simulink model "TEST_LIDAR"  (R2022b)
settings: Solver=FixedStepAuto  StartTime=0.0  StopTime=inf  FixedStep=1e-3  RelTol=1e-3  EnableMultiTasking=on
model workspace (MAT data in the model file):
  SL_ROS_VariableLengthArrays_MaxSizes : object (value not decoded)
values from neighbouring files (symbols this model uses):
  data = theClient.GetLastFrameOfData()    [FuncMotive.m]
undefined symbols (not defined in the file or in its folder): angular, carstamp, CIRCUIT, CLTF_DAMP, CLTF_FREQ, CLTF_GAIN, CONTROL, CONTROL_INI, DiscIntNeverNeededParam, INPUT, linear, MCP3201, MD25, MODEL, MODEL_INI, mpcstate, MPU60X0, MPU9250, MSG, NAV_MPC_CONTROL, OUTPUT, RCRX, SAMPLING_TIME, SYSID_INPUT, VL6180X
libraries: raspberrypiCommlib x160, simulink x89, raspberrypiNetworklib x22, ros2lib x14, dspsigattribs x14, embedlinuxBasiclib x12, ctrlSharedLib x2, mpclib x1, vrlib x1, sldrtlib x1
(part 15 of 19)

== matlab function TEST_LIDAR/SIMULATION/RC TRANSMITTER /BUS UPDATE ==
  data: CONTROL_IN input; CONTROL output Bus: CONTROL_Bus; CH_RAW input size=14
function CONTROL = RCRX_UPDATE(CONTROL_IN,CH_RAW)
%--------------------------------------------------------------
% COPY CONTROL BUS
CONTROL = CONTROL_IN;
%--------------------------------------------------------------
% SCALING PARAMETERS
% Open-loop RC scale {'COM MOTOR VOLT','DIFF MOTOR VOLT'}
OPL_RC_SCALE = CONTROL.PARAM.OPL_RC_SCALE;
% Velocity RC scale {'FORWARD VEL REF','YAW RATE REF'}
VEL_RC_SCALE = CONTROL.PARAM.VEL_RC_SCALE;
% Wall follower RC scale {'FORWARD VEL REF','WALL DIST REF'}
WFL_RC_SCALE = CONTROL.PARAM.WFL_RC_SCALE;
% Navigation RC scale {'INC POS X REF','INC POS Y REF'}
NAV_RC_SCALE = CONTROL.PARAM.NAV_RC_SCALE;
%--------------------------------------------------------------
% CHANNEL CALIBRATION
CALIB_PARAM = CONTROL.PARAM.RC_CALIB_PARAM;
CH_TRIM = CONTROL.PARAM.RC_CH_TRIM;
NUM_CH = length(CH_RAW);
CH_PU = zeros(NUM_CH,1);
CH_RAW = double(CH_RAW);
for nn = 1:NUM_CH
    CH_PU(nn) = (CALIB_PARAM(nn,1)*CH_RAW(nn) + CALIB_PARAM(nn,2)).*double(CH_RAW(nn)<CH_TRIM(nn)) + ...
                (CALIB_PARAM(nn,3)*CH_RAW(nn) + CALIB_PARAM(nn,4)).*double(CH_RAW(nn)>=CH_TRIM(nn));
end        
% Channel definition : {'COM MOTOR VOLT','DIFF MOTOR VOLT'}
%                      {'FORWARD VEL REF','YAW RATE REF'}
%                      {'FORWARD VEL REF','YAW ANGLE REF'}
%                      {'FORWARD VEL REF','WALL DIST REF'}
%                      {'INC POS X REF','INC POS Y REF'}
CH_DEF = CONTROL.PARAM.RC_CH_DEF;
% Throttle channel between 0 and 1 
% CH_PU(CH_DEF(4)) = (CH_PU(CH_DEF(4))+1)/2; 
%--------------------------------------------------------------
% TARGET DEFINITION
switch CONTROL.STATE.CONTROL_MODE 
    case 0 % OPEN LOOP
        % {'COMMON MOTOR VOLT','DIFFERENTIAL MOTOR VOLT'}
        if CONTROL.STATE.MV_TARGET_SOURCE(1)==2 % JOYSTICK
            CONTROL.TARGET.MOTOR_VOLT_CD_REF_RC(1) = CH_PU(CH_DEF(1))*OPL_RC_SCALE(1);
        end
        if CONTROL.STATE.MV_TARGET_SOURCE(2)==2 % JOYSTICK
            CONTROL.TARGET.MOTOR_VOLT_CD_REF_RC(2) = CH_PU(CH_DEF(2))*OPL_RC_SCALE(2);
        end
        if CONTROL.STATE.MV_TARGET_SOURCE(1)==3 % SWITCH
            CONTROL.TARGET.MOTOR_VOLT_CD_REF_RC(1) = CONTROL.PARAM.OPL_RC_SWITCH(1,round(2+CH_PU(5)));
        end
        if CONTROL.STATE.MV_TARGET_SOURCE(2)==3 % SWITCH
            CONTROL.TARGET.MOTOR_VOLT_CD_REF_RC(2) = CONTROL.PARAM.OPL_RC_SWITCH(2,round(2+CH_PU(6)));
        end       
    case 1 % FORWARD VELOCITY AND YAW ANGLE
        % {'FORWARD VEL REF','YAW ANGLE REF'}
        if CONTROL.STATE.FV_TARGET_SOURCE==2 % JOYSTICK
            CONTROL.TARGET.FORWARD_VEL_REF_RC = CH_PU(CH_DEF(1))*VEL_RC_SCALE(1);
        end
        if CONTROL.STATE.YA_TARGET_SOURCE==2 % JOYSTICK
            CONTROL.TARGET.YAW_ANG_REF_RC = CH_PU(CH_DEF(2))*VEL_RC_SCALE(2);
        end
        if CONTROL.STATE.FV_TARGET_SOURCE==3 % SWITCH
            CONTROL.TARGET.FORWARD_VEL_REF_RC = CONTROL.PARAM.VEL_RC_SWITCH(1,round(2+CH_PU(5)));
        end
        if CONTROL.STATE.YA_TARGET_SOURCE==3 % SWITCH
            CONTROL.TARGET.YAW_ANG_REF_RC = CONTROL.PARAM.VEL_RC_SWITCH(2,round(2+CH_PU(6)));
        end
    case 2 % FORWARD VELOCITY AND YAW RATE
        % {'FORWARD VEL REF','YAW RATE REF'}
        if CONTROL.STATE.FV_TARGET_SOURCE==2 % JOYSTICK
            CONTROL.TARGET.FORWARD_VEL_REF_RC = CH_PU(CH_DEF(1))*VEL_RC_SCALE(1);
        end
        if CONTROL.STATE.YR_TARGET_SOURCE==2 % JOYSTICK
            CONTROL.TARGET.YAW_RATE_REF_RC = CH_PU(CH_DEF(2))*VEL_RC_SCALE(2);
        end
        if CONTROL.STATE.FV_TARGET_SOURCE==3 % SWITCH
            CONTROL.TARGET.FORWARD_VEL_REF_RC = CONTROL.PARAM.VEL_RC_SWITCH(1,round(2+CH_PU(5)));
        end
        if CONTROL.STATE.YR_TARGET_SOURCE==3 % SWITCH
            CONTROL.TARGET.YAW_RATE_REF_RC = CONTROL.PARAM.VEL_RC_SWITCH(2,round(2+CH_PU(6)));
        end
    case 3 % NAVIGATION
        % {'INC POS X REF','INC POS Y REF'}
        if CONTROL.STATE.NAV_TARGET_SOURCE==2 % JOYSTICK
            CONTROL.TARGET.NAV_REF_RC(1) = CONTROL.INPUT.NAV_MO(1) + CH_PU(CH_DEF(1))*NAV_RC_SCALE;
            CONTROL.TARGET.NAV_REF_RC(2) = CONTROL.INPUT.NAV_MO(2) + CH_PU(CH_DEF(1))*NAV_RC_SCALE;
        end
        if CONTROL.STATE.NAV_TARGET_SOURCE==3 % SWITCH
            % CONTROL.TARGET.NAV_REF_RC(1) = CONTROL.INPUT.NAV_MO(1) + CONTROL.PARAM.NAV_RC_SWITCH(1,round(2+CH_PU(5)));
            % CONTROL.TARGET.NAV_REF_RC(2) = CONTROL.INPUT.NAV_MO(2) + CONTROL.PARAM.NAV_RC_SWITCH(2,round(2+CH_PU(6)));
            CONTROL.TARGET.NAV_REF_RC(1) = CONTROL.PARAM.NAV_RC_SWITCH(1,round(2+CH_PU(5)));
            CONTROL.TARGET.NAV_REF_RC(2) = CONTROL.PARAM.NAV_RC_SWITCH(2,round(2+CH_PU(6)));
        end
    case {4,5} % WALL FOLLOWER
        % {'FORWARD VEL REF','WALL DIST REF'}
        if CONTROL.STATE.FV_TARGET_SOURCE==2 % JOYSTICK
            CONTROL.TARGET.FORWARD_VEL_REF_RC = CH_PU(CH_DEF(1))*WFL_RC_SCALE(1);
        end
        % {'FORWARD VEL REF','WALL DIST REF'}
        if CONTROL.STATE.WD_TARGET_SOURCE==2 % JOYSTICK
            CONTROL.TARGET.WALL_DIST_REF_RC = 0.1 + CH_PU(CH_DEF(2))*WFL_RC_SCALE(2);
        end
        if CONTROL.STATE.FV_TARGET_SOURCE==3 % SWITCH
            CONTROL.TARGET.FORWARD_VEL_REF_RC = CONTROL.PARAM.WFL_RC_SWITCH(1,round(2+CH_PU(5)));
        end
        if CONTROL.STATE.WD_TARGET_SOURCE==3 % SWITCH
            CONTROL.TARGET.WALL_DIST_REF_RC = CONTROL.PARAM.WFL_RC_SWITCH(2,round(2+CH_PU(6)));
        end
    otherwise % FORWARD VELOCITY AND YAW RATE
        % {'FORWARD VEL REF','YAW RATE REF'}
        if CONTROL.STATE.FV_TARGET_SOURCE==2 % JOYSTICK
            CONTROL.TARGET.FORWARD_VEL_REF_RC = CH_PU(CH_DEF(1))*VEL_RC_SCALE(1);
        end
        if CONTROL.STATE.YR_TARGET_SOURCE==2 % JOYSTICK
            CONTROL.TARGET.YAW_RATE_REF_RC = CH_PU(CH_DEF(2))*VEL_RC_SCALE(1);
        end
        if CONTROL.STATE.FV_TARGET_SOURCE==3 % SWITCH
            CONTROL.TARGET.FORWARD_VEL_REF_RC = CONTROL.PARAM.VEL_RC_SWITCH(1,round(2+CH_PU(5)));
        end
        if CONTROL.STATE.YR_TARGET_SOURCE==3 % SWITCH
            CONTROL.TARGET.YAW_RATE_REF_RC = CONTROL.PARAM.VEL_RC_SWITCH(2,round(2+CH_PU(6)));
        end
end
if abs(CONTROL.TARGET.MOTOR_VOLT_CD_REF_RC(1))<0.25
    CONTROL.TARGET.MOTOR_VOLT_CD_REF_RC(1) = 0;
end
if abs(CONTROL.TARGET.MOTOR_VOLT_CD_REF_RC(2))<0.25
    CONTROL.TARGET.MOTOR_VOLT_CD_REF_RC(2) = 0;
end
if abs(CONTROL.TARGET.FORWARD_VEL_REF_RC)<0.05
    CONTROL.TARGET.FORWARD_VEL_REF_RC = 0;
end
if abs(CONTROL.TARGET.YAW_RATE_REF_RC)<0.025
    CONTROL.TARGET.YAW_RATE_REF_RC = 0;
end
%--------------------------------------------------------------
% CONTROL BUS UPDATE
% RC CHANNELS (pu): channel range [-1 1] / Throtle range (channel 4) [0 1] 
CONTROL.TARGET.RC_CH_PU = CH_PU(:);
CONTROL.TARGET.RC_CH_RAW = CH_RAW(:);

== matlab function TEST_LIDAR/HARDWARE/SENSORS/IMU MPU60X0_SPI/READ IMU/GRAVITY ROTATION ==
  data: PITCH_OFFSET input; GRAVITY_VECTOR output; GRAVITY input; VEHICLE_MODE input
function GRAVITY_VECTOR = GRAVITY_ROTATION(PITCH_OFFSET,GRAVITY,VEHICLE_MODE)
if VEHICLE_MODE
    ROTATION_MATRIX = [cos(PITCH_OFFSET) 0 -sin(PITCH_OFFSET) ; 0 1 0 ; sin(PITCH_OFFSET) 0 cos(PITCH_OFFSET)];
    GRAVITY_VECTOR = ROTATION_MATRIX*[GRAVITY ; 0 ; 0];
else
    GRAVITY_VECTOR = [0 ; 0 ; -GRAVITY];
end

== matlab function TEST_LIDAR/SIMULATION/READ ENCODER/READ_ENCODER ==
  data: MODEL input Bus: MODEL_Bus; CONTROL_IN input Bus: CONTROL_Bus; CONTROL output Bus: CONTROL_Bus
function CONTROL = READ_ENCODER(MODEL,CONTROL_IN)

%--------------------------------------------------------------
% UPDATE BUS
%--------------------------------------------------------------
CONTROL = CONTROL_IN;

%--------------------------------------------------------------
% STATE
%--------------------------------------------------------------
persistent initialize left_enc_prv right_enc_prv inc_com_ang_prv ...
           inc_dif_ang_prv inc2_com_ang_prv inc2_dif_ang_prv dif_ang ...
           dif_ang_offs left_enc_offs right_enc_offs ENC_ANG

if isempty(initialize)
    left_enc_prv = zeros(2,1);
    right_enc_prv = zeros(2,1);
    left_enc_offs = 0;
    right_enc_offs = 0;
    inc_com_ang_prv = zeros(5,1);
    inc_dif_ang_prv = zeros(5,1);
    inc2_com_ang_prv = zeros(5,1);
    inc2_dif_ang_prv = zeros(5,1);
    dif_ang = 0;
    dif_ang_offs = 0;  
    ENC_ANG = zeros(2,1);
    initialize = 1;
end

%--------------------------------------------------------------
% PARAMETERS
%--------------------------------------------------------------
% Sampling time (s)
ts = CONTROL.PARAM.SAMPLING_TIME;
% Wheel gear ratio
WHEEL_GEAR_RATIO = CONTROL.PARAM.WHEEL_GEAR_RATIO;
% Motor gear ratio
MOTOR_GEAR_RATIO = CONTROL.PARAM.MOTOR_GEAR_RATIO;
% Encoder resolution: number of pulses / revolution of main shaft
MOTOR_ENC_RES = CONTROL.PARAM.MOTOR_ENC_RES; 

%--------------------------------------------------------------
% MODEL OUTPUT READ
%--------------------------------------------------------------
WHEEL_RATE = MODEL.OUTPUT.WHEEL_RATE;
ENC_ANG = ENC_ANG + WHEEL_RATE*ts/2/pi*MOTOR_ENC_RES*MOTOR_GEAR_RATIO;
if ENC_ANG(1)>(2^31-1)
    ENC_ANG(1) = mod(ENC_ANG(1),-(2^31-1))-2;
end
if ENC_ANG(1)<-2^31
    ENC_ANG(1) = mod(ENC_ANG(1),(2^31-1))+2;
end
if ENC_ANG(2)>(2^31-1)
    ENC_ANG(2) = mod(ENC_ANG(2),-(2^31-1))-2;
end
if ENC_ANG(2)<-2^31
    ENC_ANG(2) = mod(ENC_ANG(2),(2^31-1))+2;
end
ENC_COUNT = int32(ENC_ANG);

%--------------------------------------------------------------
% ENCODER READOUT
%--------------------------------------------------------------
left_enc = double(ENC_COUNT(1));
right_enc = double(ENC_COUNT(2));
inc_right_enc = right_enc - right_enc_prv(1);
inc_left_enc = left_enc - left_enc_prv(1);
inc2_right_enc = right_enc - 2*right_enc_prv(1) + right_enc_prv(2);
inc2_left_enc = left_enc - 2*left_enc_prv(1) + left_enc_prv(2);
inc_right_ang = 360/MOTOR_ENC_RES/MOTOR_GEAR_RATIO/WHEEL_GEAR_RATIO*inc_right_enc;
inc_left_ang = 360/MOTOR_ENC_RES/MOTOR_GEAR_RATIO/WHEEL_GEAR_RATIO*inc_left_enc;
inc2_right_ang = 360/MOTOR_ENC_RES/MOTOR_GEAR_RATIO/WHEEL_GEAR_RATIO*inc2_right_enc;
inc2_left_ang = 360/MOTOR_ENC_RES/MOTOR_GEAR_RATIO/WHEEL_GEAR_RATIO*inc2_left_enc;
inc_com_ang = (inc_left_ang + inc_right_ang)/2;
inc_dif_ang = (inc_left_ang - inc_right_ang)/2;
inc2_com_ang = (inc2_left_ang + inc2_right_ang)/2;
inc2_dif_ang = (inc2_left_ang - inc2_right_ang)/2;
% Define first-order incremental encoder threshold (deg)
THR_INC_ENC_DEG = 10; 
% Define second-order incremental encoder threshold (deg)
THR_INC2_ENC_DEG = 1; 
% Check incremental limits
if (abs(inc_right_ang)>THR_INC_ENC_DEG)   || ...
   (abs(inc_left_ang)>THR_INC_ENC_DEG)    || ...
   (abs(inc2_right_ang)>THR_INC2_ENC_DEG) || ...
   (abs(inc2_left_ang)>THR_INC2_ENC_DEG)
    inc2_com_ang = mean(inc2_com_ang_prv);
    inc2_dif_ang = mean(inc2_dif_ang_prv);
    inc_com_ang = mean(inc_com_ang_prv) + inc2_com_ang;
    inc_dif_ang = mean(inc_dif_ang_prv) + inc2_dif_ang;
end
% Update differential angles
dif_ang = dif_ang + inc_dif_ang;
% Update previous values
left_enc_prv(2) = left_enc_prv(1);
right_enc_prv(2) = right_enc_prv(1);
left_enc_prv(1) = left_enc;
right_enc_prv(1) = right_enc;
inc_com_ang_prv = [inc_com_ang ; inc_com_ang_prv(1:end-1)];
inc_dif_ang_prv = [inc_dif_ang ; inc_dif_ang_prv(1:end-1)];
inc2_com_ang_prv = [inc2_com_ang ; inc2_com_ang_prv(1:end-1)];
inc2_dif_ang_prv = [inc2_dif_ang ; inc2_dif_ang_prv(1:end-1)];

%--------------------------------------------------------------
% CALIBRATION 
%--------------------------------------------------------------
ALFA_CALIB = 0.99;
if CONTROL.STATE.CURRENT_STATUS_SYS == 1  % CALIBRATION ENABLED
    dif_ang_offs  = ALFA_CALIB*dif_ang_offs  + (1-ALFA_CALIB)*dif_ang;
    left_enc_offs = ALFA_CALIB*left_enc_offs  + (1-ALFA_CALIB)*left_enc;
    right_enc_offs = ALFA_CALIB*right_enc_offs  + (1-ALFA_CALIB)*right_enc;
elseif CONTROL.STATE.CURRENT_STATUS_SYS == 0
    return
else
end 

%--------------------------------------------------------------
% ENCODER ANGLES
%--------------------------------------------------------------
CONTROL.INPUT.ENC_INC2_COM_ANG = inc2_com_ang;
CONTROL.INPUT.ENC_INC2_DIF_ANG = inc2_dif_ang;
CONTROL.INPUT.ENC_INC_COM_ANG = inc_com_ang;
CONTROL.INPUT.ENC_INC_DIF_ANG = inc_dif_ang;
CONTROL.INPUT.ENC_DIF_ANG = dif_ang-dif_ang_offs;
CONTROL.INPUT.ENC_MOTOR_ANG = 2*pi/MOTOR_ENC_RES/MOTOR_GEAR_RATIO/WHEEL_GEAR_RATIO*[left_enc-left_enc_offs right_enc-right_enc_offs]';

return

== matlab function TEST_LIDAR/SIMULATION/CAR MODEL  ==
  settings: updateMethod=DISCRETE  sampleTime=MODEL_INI.PARAM.SIM_SAMPLING_TIME
  data: STATE input; MODEL_IN input; STATE_DERIVATIVE output; MODEL output Bus: MODEL_Bus
function [STATE_DERIVATIVE,MODEL] = CAR_MODEL(STATE,MODEL_IN)
%% COPY MODEL_BUS
MODEL = MODEL_IN;

%% Reference frames
% Fixed or earth reference frame
% X,e1I - North
% Y,e2I - East
% Z,e3I - Down
% Body reference frame with origin in the center of mass
% Xb,e1B - forward axis
% Yb,e2B - right axis
% Zb,e3B - downward axis

persistent initialize TIMER
if isempty(initialize)
    TIMER = 0;
    initialize = 1;
end

%--------------------------------------------------------------
% MOTOR PARAMETERS
%--------------------------------------------------------------
% Rotor resistance (ohm)
Rm = MODEL.PARAM.MOTOR_RESISTANCE;
% Motor back-emf constant (V/rad*s)
Ke = MODEL.PARAM.MOTOR_BEMF_CONSTANT;
% Torque constant (N.m/A)
Kt = MODEL.PARAM.MOTOR_TORQUE_CONSTANT;
% Motor static torque (N. m) eje motor
Trmax = MODEL.PARAM.MOTOR_STATIC_TORQUE; 
% Viscous friction coefficient in the motor axis (N.m.s/rad)
Dm = MODEL.PARAM.MOTOR_VISCOUS_FRICTION_COEFF;
% Motor + wheel inertia in the motor axis (kg.m^2)
Im = MODEL.PARAM.MOTOR_INERTIA;
% Motor gear ratio
n1 = MODEL.PARAM.MOTOR_GEAR_RATIO;
% Converter voltage drop (V)
vc_drop = MODEL.PARAM.MOTOR_VOLT_DROP_COM;
vd_drop = MODEL.PARAM.MOTOR_VOLT_DROP_DIF;

%--------------------------------------------------------------
% CAR PARAMETERS
%--------------------------------------------------------------
% Body mass without wheels (kg)
M = MODEL.PARAM.BODY_MASS; 
% Wheel mass including the rotor (kg)
m = MODEL.PARAM.WHEEL_MASS;
% Body inertia in x-axis (kg.m^2)
Ix = MODEL.PARAM.BODY_INERTIA_X;
% Body inertia in y-axis (pitch) (kg.m^2)
Iy = MODEL.PARAM.BODY_INERTIA_Y;
% Body inertia in z-axis (kg.m^2)
Iz = MODEL.PARAM.BODY_INERTIA_Z;
% Viscous friction coefficient in x-axis (N.m.s/rad)
Dx = MODEL.PARAM.BODY_VISCOUS_FRICTION_COEFF_X;
% Viscous friction coefficient in z-axis (N.m.s/rad)
Dz = MODEL.PARAM.BODY_VISCOUS_FRICTION_COEFF_Z;
% Center of gravity distance from the wheel axis (m)
h = MODEL.PARAM.BODY_DISTANCE;
% Wheel radius (m)
R = MODEL.PARAM.WHEEL_RADIUS;
% Distance between wheels (m)
W = MODEL.PARAM.WHEEL_DISTANCE;
% Wheel gear ratio 
n2 = MODEL.PARAM.WHEEL_GEAR_RATIO; 

%--------------------------------------------------------------
% OTHER PARAMETERS
%--------------------------------------------------------------
% Gravity (m/s^2)
g = MODEL.PARAM.GRAVITY;
% Vehicle mode: / 0. CAR / 1. SELF-BALANCING VEHICLE
vmode = MODEL.PARAM.VEHICLE_MODE;
% Yaw and range sensor parameters
if vmode == 0 % CAR
    Iyaw = Iz;
    Dyaw = Dz;
    if MODEL.PARAM.WALL_FOLLOWER_MODE
        xA = MODEL.PARAM.LIDAR_2D_XA;
        yA = MODEL.PARAM.LIDAR_2D_YA;        
    else
        xA = MODEL.PARAM.RANGE_XA;
        yA = MODEL.PARAM.RANGE_YA;
    end
else % SELF-BALANCING VEHICLE
    Iyaw = Ix;
    Dyaw = Dx;
    xA = MODEL.PARAM.RANGE_ZA;
    yA = MODEL.PARAM.RANGE_YA;  
end

%--------------------------------------------------------------
% STATE VARIABLES
%--------------------------------------------------------------
% Forward velocity (m/s)
vc = STATE(1);
% Yaw rate
dShi = STATE(2);
% Yaw angle
Shi = STATE(3);
% Position in earth x-axis (m)
x = STATE(4);
% Position in earth y-axis (m)
y = STATE(5);
% Wall follower mode
if (MODEL.PARAM.CONTROL_MODE == 4) || (MODEL.PARAM.CONTROL_MODE == 5)
    % Wall distance (m)
    d_wall = STATE(6);
    % Wall angle (rad)
    Shi_wall = STATE(7);
else
    d_wall = 0;
    Shi_wall = 0;
end
% Pitch rate (rad/s)
dTheta = STATE(8);
% Pitch angle (rad)
Theta = STATE(9);
if abs(Theta)>=pi/2
    dTheta = 0;
end

%--------------------------------------------------------------
% INPUT VARIABLES
%--------------------------------------------------------------
% Motor voltages (V)
ul = MODEL.INPUT.MOTOR_VOLT(1);
ur = MODEL.INPUT.MOTOR_VOLT(2);
% Wall rotation (rad/s)
w_wall = MODEL.INPUT.WALL_RATE;

%%%%%%%%%%%%%%%%%%%%%%%%%%%%%%%%%%%%%%%%%%%%%%%%%%%%%%%%%%%%%%%%%%%%%%%%%%%
% STATE EQUATIONS
%%%%%%%%%%%%%%%%%%%%%%%%%%%%%%%%%%%%%%%%%%%%%%%%%%%%%%%%%%%%%%%%%%%%%%%%%%%
%--------------------------------------------------------------
% Common  motor voltage (V)
uc = (ul+ur)/2;
% Differential motor voltage (V)
ud = (ul-ur)/2;
%--------------------------------------------------------------
% Differential velocity of the wheels (m/s)
vd = W/2*dShi;
% (wml-wmr)/2/n2*R/W
% Common angular rate of the wheels (rad/s)
wc = vc/R;
% Differential angular rate of the wheels (rad/s)
wd = vd/R;
%--------------------------------------------------------------
% Common angular rate of the motors (rad/s)
wmc = n2*wc + dTheta/n1;
% Differential angular rate of the motors (rad/s)
wmd = n2*wd;
%--------------------------------------------------------------
% Motor rate 
wml = wmc + wmd;
wmr = wmc - wmd;
% wmc = (wmr+wml)/2;
% wmd = (wml-wmr)/2
%--------------------------------------------------------------
% Motor equations
el = Ke*wml;
er = Ke*wmr;
vl_drop = sign(ul-el)*(vc_drop+vd_drop);
vr_drop = sign(ur-er)*(vc_drop-vd_drop);
if abs(ul-el)<vl_drop
    vl_drop = 0;    
end
if abs(ur-er)<vr_drop
    vr_drop = 0;
end
% Currents
il = (ul-vl_drop-el)/Rm;
ir = (ur-vr_drop-er)/Rm;
% ic = (il+ir)/2;
% id = (il-ir)/2;
% dil = (ul - el - Rm*il)/Lm;
% dir = (ur - er - Rm*ir)/Lm;
% Motor torques
Tml = Kt*il;
Tmr = Kt*ir;
Tmc = (Tml+Tmr)/2;
Tmd = (Tml-Tmr)/2;
%--------------------------------------------------------------
% Static friction torques
Trl_lim = Tml*(abs(Tml)<Trmax) - Trmax*(Tml<=-Trmax) + Trmax*(Tml>=Trmax);
Trl = Trl_lim*(abs(wml)==0) + Trmax*sign(wml)*(abs(wml)>0);
Trr_lim = Tmr*(abs(Tmr)<Trmax) - Trmax*(Tmr<=-Trmax) + Trmax*(Tmr>=Trmax);
Trr = Trr_lim*(abs(wmr)==0) + Trmax*sign(wmr)*(abs(wmr)>0);
Trc = (Trl+Trr)/2;
Trd = (Trl-Trr)/2;
%--------------------------------------------------------------
% Viscous friction torques
Tdl = Dm*wml;
Tdr = Dm*wmr;
Tdc = (Tdr+Tdl)/2;
Tdd = (Tdl-Tdr)/2;
%--------------------------------------------------------------
% Total motor torque
% Tl = Tml - Tdl - Trl - Frl*R/n2;
% Tr = Tmr - Tdr - Trr - Frr*R/n2;
%--------------------------------------------------------------
% Motor angular accelerations
% dwml = Tl/Im = (Tml-Tdl-Trl-Frl*R/n2)/Im
% dwmr = Tr/Im = (Tmr-Tdr-Trr-Frr*R/n2)/Im
%--------------------------------------------------------------
% Friction body forces
% Frl = n2/R*(Tml-Tdl-Trl-Im*dwml)
% Frr = n2/R*(Tmr-Tdr-Trr-Im*dwmr)
%--------------------------------------------------------------
if vmode == 0
    %--------------------------------------------------------------
    % Translation equation in x-axis (CAR)
    % Frl + Frr = (M+2*m)*dvc
    % 2*n2/R*(Tmc-Tdc-Trc) = (M+2*m+2*(n2/R)^2*Im)*dvc
    %---------------------------------------------------------    %--------------------------------------------------------------
    % Computation of dvc (CAR)
    dvc = 2*n2/R*(Tmc-Tdc-Trc)/(M+2*m+2*(n2/R)^2*Im);
    d2Theta = 0;
    % (M+2*m+2*(n2/R)^2*Im)*dvc + 2*n2^2/R^2*(Dm+Kt*Ke/Rm)*vc = 2*n2*Kt/R/Rm*uc
    % Tv*dvc + vc = Kv*uc
    % Kv = 2*n2*Kt/R/Rm/(2*(n2/R)^2*(Dm+Kt*Ke/Rm))
    % Tv = (M+2*m+2*(n2/R)^2*Im)/(2*(n2/R)^2*(Dm+Kt*Ke/Rm))
    %--------------------------------------------------------------
else
    %--------------------------------------------------------------
    % Translation equation in x-axis (c)
    % Frl + Frr = (M+2*m)*dvc  - M*h*cos(Theta)*d2Theta + M*h*sin(Theta)*dTheta^2
    % 2*n2/R*(Tmc-Tdc-Trc) - M*h*sin(Theta)*dTheta^2 =
    %    = (M+2*m+2*(n2/R)^2*Im)*dvc  - (M*h*cos(Theta)-2*n2/n1/R*Im)*d2Theta
    %--------------------------------------------------------------
    % Chassis reaction force Nx (SELF-BALANCING VEHICLE)
    % Nx - M*g*sin(Theta) = M*cos(Theta)*dvc - M*h*d2Theta
    % h*Nx + 2*Tc = Iy*d2Theta (2/30*Tc is ignored)
    % Nx = M*cos(Theta)*dvc - M*h*d2Theta + M*g*sin(Theta)
    % M*g*h*sin(Theta) + M*h*cos(Theta)*dvc - M*h^2*d2Theta + 2*Tc = Iy*d2Theta
    % 2*Tc + M*g*h*sin(Theta) = -M*h*cos(Theta)*dvc + (Iy+M*h^2)*d2Theta
    % M*g*h*sin(Theta) = -(M*h*cos(Theta)+2/R*Im)*dvc + (Iy+M*h^2-2*Im/n1^2)*d2Theta
    %--------------------------------------------------------------
    % Computation of dvc and d2Theta (SELF-BALANCING VEHICLE)
    matA = [       M+2*m+2*(n2/R)^2*Im      -(M*h*cos(Theta)-2*n2/n1/R*Im)
             -(M*h*cos(Theta)+2/R*Im)        Iy+M*h^2-2*Im/n1^2      ];
    matB = [   2*n2/R*(Tmc-Tdc-Trc)-M*h*dTheta^2*sin(Theta)
                               M*g*h*sin(Theta) ];
    aux = matA\matB;
    dvc = aux(1);
    d2Theta = aux(2);
    %--------------------------------------------------------------
end
%--------------------------------------------------------------
% Rotation equation in yaw-axis
% Frl - Frr = 2*n2/R*(Tmd-Tdd-Trd-Im*dwmd)
% Torque in yaw-axis (earth reference-frame)
% Tz = (Frl-Frr)*W/2 - Dyaw*dShi
% Iyaw*d2Shi = W/2*(Frl-Frr) - Dyaw*dShi
% Iyaw*d2Shi = n2*W/R*(Tmd-Tdd-Trd-Im*dwmd) - Dyaw*dShi
% wmd = n2*wd = n2/R*vd = n2*W/2/R*dShi
% dwmd = W/R/2*d2Shi
% Iyaw*d2Shi = n2*W/R*(Tmd-Tdd-Trd-Im*n2*W/R/2*d2Shi) - Dyaw*dShi
% (Iyaw+(n2*W/R)^2/2*Im)*d2Shi = n2*W/R*(Tmd-Tdd-Trd) - Dyaw*dShi
d2Shi = 1/(Iyaw+(n2*W/R)^2/2*Im)*(n2*W/R*(Tmd-Tdd-Trd) - Dyaw*dShi);
% (Iyaw+(n2*W/R)^2/2*Im)*d2Shi + Dyaw*dShi + n2*W/R*Tdd  = n2*W/R/Rm*Kt*(ud-ed)
% (Iz+n2*(W/R)^2/2*Im)*d2Shi + Dz*dShi + n2^2/R^2*W^2/2*Dm*dShi + n2^2/R^2*W^2/2*Kt*Ke/Rm*dShi = n2*W/R/Rm*Kt*ud
% Kw = n2/R*W*Kt/Rm/(Dyaw+n2^2/R^2*W^2/2*(Dm+Kt*Ke/Rm))
% Tw = (Iyaw+(n2*W/R)^2/2*Im)/(Dyaw+n2^2/R^2*W^2/2*(Dm+Kt*Ke/Rm))
%---------------------------------------------------------
% Earth velocity
vx = vc*cos(Shi);
vy = vc*sin(Shi);
vz = 0;
vxyz = [vx vy vz]';
dvx = dvc*cos(Shi) - vc*sin(Shi)*dShi;
dvy = dvc*sin(Shi) + vc*cos(Shi)*dShi;
dvz = 0;
dvxyz = [dvx dvy dvz]';
%--------------------------------------------------------------
% Wall distance derivative
dd_wall = 0;
dShi_wall = 0;
% Wall follower model
if (MODEL.PARAM.CONTROL_MODE == 4) || (MODEL.PARAM.CONTROL_MODE == 5)
    dShi_wall = dShi - w_wall; 
    dd_wall = -(vc-dShi_wall*yA)*sin(Shi_wall) - dShi_wall*xA*cos(Shi_wall);
end
if vmode && TIMER<1
    dvc = 0; d2Shi = 0; dShi = 0; vx = 0; vy = 0; dd_wall = 0; 
    dShi_wall = 0; d2Theta = 0; dTheta = 0; dvxyz = zeros(3,1);
    TIMER = TIMER + MODEL.PARAM.SIM_SAMPLING_TIME;
end

%%%%%%%%%%%%%%%%%%%%%%%%%%%%%%%%%%%%%%%%%%%%%%%%%%%%%%%%%%%%%%%%%%%%%%%%%%%
STATE_DERIVATIVE = [dvc ; d2Shi ; dShi ; vx ; vy ; dd_wall ; dShi_wall ; ...
                    d2Theta ; dTheta];
%%%%%%%%%%%%%%%%%%%%%%%%%%%%%%%%%%%%%%%%%%%%%%%%%%%%%%%%%%%%%%%%%%%%%%%%%%%

%%%%%%%%%%%%%%%%%%%%%%%%%%%%%%%%%%%%%%%%%%%%%%%%%%%%%%%%%%%%%%%%%%%%%%%%%%%
% OUTPUT BUS
%%%%%%%%%%%%%%%%%%%%%%%%%%%%%%%%%%%%%%%%%%%%%%%%%%%%%%%%%%%%%%%%%%%%%%%%%%%
% COMPUTATION OF EULER ANGLES, RATES & MATRICES 
if vmode == 0 % CAR
    % Roll angle (rad)
    Phi_car = 0;
    % Roll rate (rad/s)
    dPhi_car = 0;
    % Roll acceleration (rad/s^2)
    d2Phi_car = 0;
    % Pitch angle (rad)
    Theta_car = Theta;
    % Pitch rate (rad/s)
    dTheta_car = dTheta;
    % Pitch acceleration (rad/s^2)
    d2Theta_car = d2Theta;    
    % Yaw angle (rad)
    Shi_car = Shi;
    % Yaw rate (rad/s)
    dShi_car = dShi;
    % Yaw acceleration (rad/s^2)
    d2Shi_car = d2Shi;    
else % SELF-BALANCING VEHICLE
    % Roll angle (rad)
    Phi_car = -Shi;
    % Roll rate (rad/s)
    dPhi_car = -dShi;
    % Roll acceleration (rad/s^2)
    d2Phi_car = -d2Shi;
    % Pitch angle (rad)
    Theta_car = Theta+pi/2-MODEL.PARAM.IMU_PITCH_OFFSET;
    % Pitch rate (rad/s)
    dTheta_car = dTheta;
    % Pitch acceleration (rad/s^2)
    d2Theta_car = d2Theta; 
    % Yaw angle (rad)
    Shi_car = 0;
    % Yaw rate (rad/s)
    dShi_car = 0;
    % Yaw acceleration (rad/s^2)
    d2Shi_car = 0;    
end
MODEL.OUTPUT.EULER_ANG = [Phi_car ; Theta_car ; Shi_car];
MODEL.OUTPUT.EULER_RATE = [dPhi_car ; dTheta_car ; dShi_car];
MODEL.OUTPUT.EULER_RATE_DER = [d2Phi_car ; d2Theta_car ; d2Shi_car];
MODEL.OUTPUT.matDCM_BE = ...
 [ cos(Theta_car)*cos(Shi_car) sin(Phi_car)*sin(Theta_car)*cos(Shi_car)-cos(Phi_car)*sin(Shi_car)  cos(Phi_car)*sin(Theta_car)*cos(Shi_car)+sin(Phi_car)*sin(Shi_car)
   sin(Shi_car)*cos(Theta_car) sin(Phi_car)*sin(Theta_car)*sin(Shi_car)+cos(Phi_car)*cos(Shi_car)  cos(Phi_car)*sin(Theta_car)*sin(Shi_car)-sin(Phi_car)*cos(Shi_car)
  -sin(Theta_car)          sin(Phi_car)*cos(Theta_car)                             cos(Phi_car)*cos(Theta_car)                           ];
MODEL.OUTPUT.matEULER = [ 1     0         -sin(Theta_car)
                          0  cos(Phi_car) sin(Phi_car)*cos(Theta_car)
                          0 -sin(Phi_car) cos(Phi_car)*cos(Theta_car) ];
% matEuler = [ 1     0         -sin(Theta)
%              0  cos(Phi) sin(Phi)*cos(Theta)
%              0 -sin(Phi) cos(Phi)*cos(Theta) ]
MODEL.OUTPUT.matEULER_DER = [ 0          0                         -cos(Theta_car)*dTheta_car
                              0 -sin(Phi_car)*dPhi_car   cos(Phi_car)*cos(Theta_car)*dPhi_car-sin(Phi_car)*sin(Theta_car)*dTheta_car
                              0 -cos(Phi_car)*dPhi_car  -sin(Phi_car)*cos(Theta_car)*dPhi_car-cos(Phi_car)*sin(Theta_car)*dTheta_car ];
% wxyz = matEuler*dEuler;
MODEL.OUTPUT.BODY_RATE = MODEL.OUTPUT.matEULER*MODEL.OUTPUT.EULER_RATE;
% dwxyz = matEuler_der*dEuler + matEuler*d2Euler
MODEL.OUTPUT.BODY_RATE_DER = MODEL.OUTPUT.matEULER*MODEL.OUTPUT.EULER_RATE_DER + ...
                             MODEL.OUTPUT.matEULER_DER*MODEL.OUTPUT.EULER_RATE;
MODEL.OUTPUT.EARTH_VEL = vxyz;
MODEL.OUTPUT.EARTH_POS = [x ; y ; 0];
MODEL.OUTPUT.EARTH_VEL_DER = dvxyz;
MODEL.OUTPUT.BODY_VEL_DER = MODEL.OUTPUT.matDCM_BE'*dvxyz;
MODEL.OUTPUT.FORWARD_VEL = vc;
MODEL.OUTPUT.PITCH_ANG = Theta;
MODEL.OUTPUT.YAW_ANG = Shi;
MODEL.OUTPUT.PITCH_RATE = dTheta;
MODEL.OUTPUT.YAW_RATE = dShi;
MODEL.OUTPUT.MOTOR_VOLT_CD = [uc ; ud];
MODEL.OUTPUT.MOTOR_CURRENT = [il ; ir];
MODEL.OUTPUT.MOTOR_RATE = [wml ; wmr];
MODEL.OUTPUT.WHEEL_RATE = MODEL.OUTPUT.MOTOR_RATE/n2;
MODEL.OUTPUT.WALL_DIST = d_wall;
MODEL.OUTPUT.WALL_ANG = Shi_wall;

return

== matlab function TEST_LIDAR/CONTROL/ADAPTIVE CONTROL STR/PI DESIGN ==
  data: PARAM input; K_out output; Ti_out output; b_out output; FLAG_ADPT_out output; CONTROL input Bus: CONTROL_Bus
function [K_out,Ti_out,b_out,FLAG_ADPT_out] = PI_DESIGN(PARAM,CONTROL)

%--------------------------------------------------------------
% PERSISTENT VARIABLES
%--------------------------------------------------------------
persistent TIMER K Ti b FLAG_ADPT initialize
if isempty(initialize)
    TIMER = 0;
    K = CONTROL.PARAM.FORWARD_VEL_PID.K;
    Ti = CONTROL.PARAM.FORWARD_VEL_PID.Ti;
    b = CONTROL.PARAM.FORWARD_VEL_PID.b;
    FLAG_ADPT = false;
    initialize = 1;
end

TIMER = TIMER + CONTROL.PARAM.SAMPLING_TIME;
if TIMER < 2
    K_out = K;
    Ti_out = Ti;
    b_out = b;
    FLAG_ADPT_out = FLAG_ADPT; 
    return
else
    TIMER = 0;
end

%% TRANSFER FUNCTION COEFFICIENTS
a1 = -PARAM(1);
a2 = -PARAM(2);
b0 = PARAM(3);

%% SPECIFICATIONS
wn = 10;
seta = 0.7;

%% CONTROL PARAMETERS
tao = a2/(a1-2*a2*seta*wn);
K = (a2*wn^2+2*a2*seta*wn/tao-1)/b0;
Ti = b0*K*tao/a2/wn^2;
b = tao/Ti;
FLAG_ADPT = false;
if K>0 && Ti>0 && tao>0 && b>0
    FLAG_ADPT = true;
end
K_out = K;
Ti_out = Ti;
b_out = b;
FLAG_ADPT_out = FLAG_ADPT;

== matlab function TEST_LIDAR/GAZEBO SIMULATION/SENSORS/READ IMU/GRAVITY ROTATION ==
  data: PITCH_OFFSET input; GRAVITY_VECTOR output; GRAVITY input; VEHICLE_MODE input
function GRAVITY_VECTOR = GRAVITY_ROTATION(PITCH_OFFSET,GRAVITY,VEHICLE_MODE)
if VEHICLE_MODE
    ROTATION_MATRIX = [cos(PITCH_OFFSET) 0 -sin(PITCH_OFFSET) ; 0 1 0 ; sin(PITCH_OFFSET) 0 cos(PITCH_OFFSET)];
    GRAVITY_VECTOR = ROTATION_MATRIX*[GRAVITY ; 0 ; 0];
else
    GRAVITY_VECTOR = [0 ; 0 ; -GRAVITY];
end

== matlab function TEST_LIDAR/GAZEBO SIMULATION/SENSORS/READ IMU/IMU CALIBRATION ==
  data: CONTROL_IN input; ACCEL input; ACCEL_FILT input; ACCEL_MEAN input; ACCEL_MEAN_FILT input; GYRO input; GYRO_FILT input; GYRO_MEAN input; GYRO_MEAN_FILT input; ACCEL_CALIB input; ALFA_CALIB input; ACCEL_OFFS_IN input; GYRO_OFFS_IN input; CONTROL output Bus: CONTROL_Bus; ACCEL_OFFS_OUT output; GYRO_OFFS_OUT output; GRAVITY_VECTOR input
function [CONTROL,ACCEL_OFFS_OUT,GYRO_OFFS_OUT] = IMU_CALIBRATION(CONTROL_IN,...
                       ACCEL,ACCEL_FILT,ACCEL_MEAN,ACCEL_MEAN_FILT,...
                       GYRO,GYRO_FILT,GYRO_MEAN,GYRO_MEAN_FILT,...
                       ACCEL_CALIB,ALFA_CALIB,ACCEL_OFFS_IN,GYRO_OFFS_IN,GRAVITY_VECTOR)
                        
%--------------------------------------------------------------
% COPY CONTROL BUS
%--------------------------------------------------------------
CONTROL = CONTROL_IN;

%--------------------------------------------------------------
% IMU ORIENTATION
%--------------------------------------------------------------
% ACCEL = [0 0 1 ; 1 0 0 ; 0 1 0]*ACCEL;
% GYRO = [0 0 1 ; 1 0 0 ; 0 1 0]*GYRO;
ACCEL_MEAN = [0 0 1 ; 1 0 0 ; 0 1 0]*ACCEL_MEAN;
GYRO_MEAN = [0 0 1 ; 1 0 0 ; 0 1 0]*GYRO_MEAN;
% ACCEL_FILT = [0 0 1 ; 1 0 0 ; 0 1 0]*ACCEL_FILT;
% GYRO_FILT = [0 0 1 ; 1 0 0 ; 0 1 0]*GYRO_FILT;
ACCEL_MEAN_FILT = [0 0 1 ; 1 0 0 ; 0 1 0]*ACCEL_MEAN_FILT;
GYRO_MEAN_FILT = [0 0 1 ; 1 0 0 ; 0 1 0]*GYRO_MEAN_FILT;

%--------------------------------------------------------------
% CALIBRATION 
%--------------------------------------------------------------
if CONTROL.STATE.CURRENT_STATUS_SYS == 1  % CALIBRATION ENABLED
    if ACCEL_CALIB % ACCELEROMETER CALIBRATION ENABLED
        ACCEL_OFFS_OUT = ALFA_CALIB*ACCEL_OFFS_IN + (1-ALFA_CALIB)*(ACCEL_MEAN_FILT-GRAVITY_VECTOR);
    else
        ACCEL_OFFS_OUT = ACCEL_OFFS_IN;
    end
    GYRO_OFFS_OUT  = ALFA_CALIB*GYRO_OFFS_IN  + (1-ALFA_CALIB)*GYRO_MEAN_FILT;
else % END OF CALIBRATION
    ACCEL_OFFS_OUT = ACCEL_OFFS_IN;  
    GYRO_OFFS_OUT  = GYRO_OFFS_IN;
    % ACCEL = ACCEL - ACCEL_OFFS_OUT;
    % GYRO = GYRO - GYRO_OFFS_OUT;
    ACCEL_MEAN = ACCEL_MEAN - ACCEL_OFFS_OUT;
    GYRO_MEAN = GYRO_MEAN - GYRO_OFFS_OUT;
    % ACCEL_FILT = ACCEL_FILT - ACCEL_OFFS_OUT;
    % GYRO_FILT = GYRO_FILT - GYRO_OFFS_OUT;
    ACCEL_MEAN_FILT = ACCEL_MEAN_FILT - ACCEL_OFFS_OUT;
    GYRO_MEAN_FILT = GYRO_MEAN_FILT - GYRO_OFFS_OUT;
end

%--------------------------------------------------------------
% IMU BUS UPDATE
%--------------------------------------------------------------
% CONTROL.INPUT.IMU_ACCEL = ACCEL;
% CONTROL.INPUT.IMU_GYRO = GYRO;
CONTROL.INPUT.IMU_ACCEL_MEAN = ACCEL_MEAN;
CONTROL.INPUT.IMU_GYRO_MEAN = GYRO_MEAN;
% CONTROL.INPUT.IMU_ACCEL_FILT = ACCEL_FILT;
% CONTROL.INPUT.IMU_GYRO_FILT = GYRO_FILT;
CONTROL.INPUT.IMU_ACCEL_MEAN_FILT = ACCEL_MEAN_FILT;
CONTROL.INPUT.IMU_GYRO_MEAN_FILT = GYRO_MEAN_FILT;

return

== matlab function TEST_LIDAR/HARDWARE/COMMUNICATIONS/TCP//IP NAV/NAV RX ==
  data: CONTROL_IN input; PAYLOAD input; CONTROL output Bus: CONTROL_Bus; STATUS input
function CONTROL  = NAV_DECODER(CONTROL_IN,PAYLOAD,STATUS)
% Initialization
CONTROL = CONTROL_IN;
%%%%%%%%%%%%%%%%%%%%%%%%%%%%%%%%%%%%%%%%%%%%%%%%%%%%%%%%%%%%%%%%%%%%%%%%%%%
% MCS MESSAGES
%%%%%%%%%%%%%%%%%%%%%%%%%%%%%%%%%%%%%%%%%%%%%%%%%%%%%%%%%%%%%%%%%%%%%%%%%%%
% WRITE IN THE CONTROL BUS
if STATUS==1
    CONTROL.INPUT.NAV_EARTH_POS(1) = double(typecast(PAYLOAD(4:-1:1),'single'));
    CONTROL.INPUT.NAV_EARTH_POS(2) = double(typecast(PAYLOAD(8:-1:5),'single'));
    CONTROL.INPUT.NAV_EARTH_POS(3) = double(typecast(PAYLOAD(12:-1:9),'single'));
    CONTROL.INPUT.NAV_EULER_ANG(1) = double(typecast(PAYLOAD(16:-1:13),'single'));
    CONTROL.INPUT.NAV_EULER_ANG(2) = double(typecast(PAYLOAD(20:-1:17),'single'));
    CONTROL.INPUT.NAV_EULER_ANG(3) = double(typecast(PAYLOAD(24:-1:21),'single'));
    if CONTROL.STATE.CURRENT_STATUS_SYS>1
        CONTROL.INPUT.NAV_EARTH_POS = CONTROL.INPUT.NAV_EARTH_POS - CONTROL.PARAM.NAV_EARTH_POS_OFFS;
        CONTROL.INPUT.NAV_EULER_ANG = CONTROL.INPUT.NAV_EULER_ANG - CONTROL.PARAM.NAV_EULER_ANG_OFFS;
    end
end
% UNWRAPPING
aux1 = CONTROL.INPUT.NAV_EULER_ANG(3);
aux2 = CONTROL.INPUT.YAW_ANG;
INC_ANG = zeros(41,1);
INC_ANG(1) = aux1-aux2;
for ii = 1:20
    INC_ANG(2*ii)   = aux1-aux2-2*ii*pi;
    INC_ANG(2*ii+1) = aux1-aux2+2*ii*pi;
end
[~,ind] = min(abs(INC_ANG));
NAV_YAW_ANG = aux2 + INC_ANG(ind);
CONTROL.INPUT.NAV_EULER_ANG(3) = NAV_YAW_ANG;
%%%%%%%%%%%%%%%%%%%%%%%%%%%%%%%%%%%%%%%%%%%%%%%%%%%%%%%%%%%%%%%%%%%%%%%%%%%


return

== matlab function TEST_LIDAR/HARDWARE/SENSORS/IMU MPU60X0_SPI/READ FIFO/FIFO_PROCESSING ==
  data: CONTROL_IN input Bus: CONTROL_Bus; FIFO_DATA input; CONTROL_OUT output Bus: CONTROL_Bus; FIFO_LENGTH input; RAW_GYRO_MEAN_OUT output; RAW_ACCEL_MEAN_OUT output; ACCEL_SSF input; GYRO_SSF input; ACCEL_FIFO output; GYRO_FIFO output
function [CONTROL_OUT,RAW_GYRO_MEAN_OUT,RAW_ACCEL_MEAN_OUT,ACCEL_FIFO,GYRO_FIFO] = FIFO_PROCESSING(CONTROL_IN,FIFO_DATA,FIFO_LENGTH,ACCEL_SSF,GYRO_SSF)

%% INITIALIZATION
FIFO_DATA = FIFO_DATA(:);
AUX = single(zeros(3,FIFO_LENGTH));
GRAVITY = CONTROL_IN.PARAM.GRAVITY;
GYRO_FIFO = zeros(30,1,'single');
ACCEL_FIFO = zeros(30,1,'single');

%% GYROSCOPE
for nn = 1:FIFO_LENGTH
    ii = 2*nn;
    AUX(:,nn) = single(FIFO_DATA(3*(ii-1)+1:3*ii));
end
RAW_GYRO_MEAN = sum(AUX,2)/single(FIFO_LENGTH);
RAW_GYRO = AUX(:,end);
GYRO_FIFO(1:30) = [AUX(1,:) AUX(2,:) AUX(3,:)]'/GYRO_SSF*pi/180;


%% ACCELEROMETER
for nn = 1:FIFO_LENGTH
    ii = 2*nn-1;
    AUX(:,nn) = single(FIFO_DATA(3*(ii-1)+1:3*ii));
end
RAW_ACCEL_MEAN = sum(AUX,2)/single(FIFO_LENGTH);
RAW_ACCEL = AUX(:,end);
ACCEL_FIFO(1:30) = [AUX(1,:) AUX(2,:) AUX(3,:)]'/ACCEL_SSF*GRAVITY;

%% SENSOR BUS UPDATE
CONTROL_OUT = CONTROL_IN;
CONTROL_OUT.INPUT.IMU.RAW_GYRO = int16(RAW_GYRO);
CONTROL_OUT.INPUT.IMU.RAW_ACCEL = int16(RAW_ACCEL);
RAW_GYRO_MEAN_OUT = int16(RAW_GYRO_MEAN);
RAW_ACCEL_MEAN_OUT = int16(RAW_ACCEL_MEAN);

== matlab function TEST_LIDAR/HARDWARE/COMMUNICATIONS/TCP//IP LIDAR/NAV RX ==
  data: CONTROL_IN input; PAYLOAD input; CONTROL output Bus: CONTROL_Bus; STATUS input
function CONTROL  = NAV_DECODER(CONTROL_IN,PAYLOAD,STATUS)
% Initialization
CONTROL = CONTROL_IN;
%%%%%%%%%%%%%%%%%%%%%%%%%%%%%%%%%%%%%%%%%%%%%%%%%%%%%%%%%%%%%%%%%%%%%%%%%%%
% MCS MESSAGES
%%%%%%%%%%%%%%%%%%%%%%%%%%%%%%%%%%%%%%%%%%%%%%%%%%%%%%%%%%%%%%%%%%%%%%%%%%%
% WRITE IN THE CONTROL BUS
if STATUS==1
    for nn = 1:20
        CONTROL.INPUT.LIDAR_2D(nn,1) = double(typecast(PAYLOAD(8*nn-4:-1:8*(nn-1)+1),'single'));
        CONTROL.INPUT.LIDAR_2D(nn,2) = double(typecast(PAYLOAD(8*nn:-1:8*nn-3),'single'));
    end
end
%%%%%%%%%%%%%%%%%%%%%%%%%%%%%%%%%%%%%%%%%%%%%%%%%%%%%%%%%%%%%%%%%%%%%%%%%%%


return

== matlab function TEST_LIDAR/HARDWARE/SENSORS/IMU MPU60X0_SPI/READ TEMP/IMU SCALING ==
  data: CONTROL_IN input; CONTROL_OUT output Bus: SENSOR_Bus; TEMP_SSF input; TEMP_OFFS input
function CONTROL_OUT = IMU_SCALING(CONTROL_IN,TEMP_SSF,TEMP_OFFS)

%% INPUT
CONTROL_OUT = CONTROL_IN;
RAW_TEMP = CONTROL_OUT.IMU.TEMP;

%% TEMP SCALING
SCALED_TEMP = int16(100*(single(RAW_TEMP)/TEMP_SSF + TEMP_OFFS)); % ºC/100
TEMP = single(100*SCALED_TEMP);

%% IMU BUS UPDATE
CONTROL_OUT.INPUT.IMU.SCALED_TEMP = SCALED_TEMP;
CONTROL_OUT.INPUT.IMU.TEMP = TEMP;

== matlab function TEST_LIDAR/HARDWARE/COMMUNICATIONS/TCP//IP MCS/MCS RX ==
  data: CONTROL_IN input; PAYLOAD input; CONTROL output Bus: CONTROL_Bus; STATUS input
function CONTROL = MCS_DECODER(CONTROL_IN,PAYLOAD,STATUS)
% Initialization
CONTROL = CONTROL_IN;
%%%%%%%%%%%%%%%%%%%%%%%%%%%%%%%%%%%%%%%%%%%%%%%%%%%%%%%%%%%%%%%%%%%%%%%%%%%
% MCS MESSAGES
%%%%%%%%%%%%%%%%%%%%%%%%%%%%%%%%%%%%%%%%%%%%%%%%%%%%%%%%%%%%%%%%%%%%%%%%%%%

% CRC    
CRC_VALUE=uint16(65535);
for nn=1:24
    TMP=bitxor(uint16(PAYLOAD(nn)),bitand(CRC_VALUE,uint16(255)));
    TMP4=bitand(bitshift(TMP,4),uint16(255));
    TMP=bitxor(TMP,TMP4);
    TMP8=bitshift(TMP,8);
    TMP3=bitshift(TMP,3);
    TMP_4=bitshift(TMP,-4);
    CRC_VALUE=bitxor(bitshift(CRC_VALUE,-8),bitxor(TMP8,bitxor(TMP3,TMP_4)));
    CRC_VALUE=bitand(CRC_VALUE,uint16(65535));
end
CRC1=uint8(bitand(CRC_VALUE,uint16(255)));
CRC2=uint8(bitand(bitshift(CRC_VALUE,-8),uint16(255)));
% CRC checking
if (CRC1 == PAYLOAD(MESSAGE_LEN-1))  && (CRC2 == PAYLOAD(MESSAGE_LEN))
    % WRITE IN THE CONTROL BUS
    CONTROL.INPUT.MCS_EARTH_POS(1) = double(typecast(PAYLOAD(1:4),'single'));
    CONTROL.INPUT.MCS_EARTH_POS(2) = double(typecast(PAYLOAD(5:8),'single'));
    CONTROL.INPUT.MCS_EARTH_POS(3) = double(typecast(PAYLOAD(9:12),'single'));
    CONTROL.INPUT.MCS_EULER_ANG(1) = double(typecast(PAYLOAD(13:16),'single'));
    CONTROL.INPUT.MCS_EULER_ANG(2) = double(typecast(PAYLOAD(17:20),'single'));
    CONTROL.INPUT.MCS_EULER_ANG(3) = double(typecast(PAYLOAD(21:24),'single'));

    % UNWRAPPING
    aux1 = CONTROL.INPUT.MCS_EULER_ANG(3);
    aux2 = CONTROL.TARGET.YAW_ANG_REF;
    INC_ANG = zeros(41,1);
    INC_ANG(1) = aux1-aux2;
    for ii = 1:20
        INC_ANG(2*ii)   = aux1-aux2-2*ii*pi;
        INC_ANG(2*ii+1) = aux1-aux2+2*ii*pi;
    end
    [~,ind] = min(abs(INC_ANG));
    NAV_YAW_ANG = aux2 + INC_ANG(ind);
    CONTROL.INPUT.MCS_EULER_ANG(3) = NAV_YAW_ANG;

    % POSITION CORRECTION
    % rv = rm + rc*exp(Shi*j)
    % xv = xm + xc*cos(Shi);
    % yv = ym + yc*sin(Shi);
    CONTROL.INPUT.MCS_EARTH_POS(1) = CONTROL.INPUT.MCS_EARTH_POS(1) - CONTROL.PARAM.NAV_CENTER_POS(1)*cos(CONTROL.INPUT.MCS_EULER_ANG(3));
    CONTROL.INPUT.MCS_EARTH_POS(2) = CONTROL.INPUT.MCS_EARTH_POS(2) - CONTROL.PARAM.NAV_CENTER_POS(2)*sin(CONTROL.INPUT.MCS_EULER_ANG(3));

    % INITIAL POSITION COMPENSATION
    if CONTROL.STATE.CURRENT_STATUS_SYS>1
        CONTROL.INPUT.MCS_EARTH_POS = CONTROL.INPUT.MCS_EARTH_POS - CONTROL.PARAM.MCS_EARTH_POS_OFFS;
        CONTROL.INPUT.MCS_EULER_ANG = CONTROL.INPUT.MCS_EULER_ANG - CONTROL.PARAM.MCS_EULER_ANG_OFFS;
    end
    
end


return

== matlab function TEST_LIDAR/NAVIGATION/NAVIGATION TARGETS/TRAJECTORY PLANNER (POLYNOMIAL IN Vx & Vy) ==
  data: CONTROL_IN input Bus: CONTROL_Bus; CONTROL output Bus: CONTROL_Bus
function CONTROL = MPC_TARGET_UPDATE(CONTROL_IN)

%--------------------------------------------------------------
% COPY CONTROL BUS
%--------------------------------------------------------------
CONTROL = CONTROL_IN;

%--------------------------------------------------------------
% DISABLING TARGET UPDATE
%--------------------------------------------------------------
% CONTROL_STATUS
% / 0. INITIALIZATION     / 1. ESTIMATION    / 2. ACTIVE CONTROL
if CONTROL.STATE.CONTROL_STATUS < 2  % INITIALIZATION    
    return
end

%--------------------------------------------------------------
% TIME MANAGEMENT
%--------------------------------------------------------------
% Sampling time 
ts = CONTROL.PARAM.SAMPLING_TIME;
% Trajectory update time 
tc = 10*ts;
persistent initialize TIMER
if isempty(initialize)
    TIMER = 0;
    initialize = 1;
end
TIMER = TIMER + ts;
if TIMER > tc-ts/2
    TIMER = 0;
    return
end

%--------------------------------------------------------------
% PARAMETERS
%--------------------------------------------------------------
% Maximun velocity magnitude 
VEL_MAG_MAX = CONTROL.PARAM.VEL_MAG_MAX;
% Prediction horizon (<= prediction horizon in mpcDesigner)
P = 20;
% Circular outline radius
% WP_R = CONTROL.PARAM.WP_R;

%--------------------------------------------------------------
% MEASUREMENTS AND STATE
%--------------------------------------------------------------
VEL_MAG = CONTROL.INPUT.FORWARD_VEL;
VEL_ANG = CONTROL.INPUT.YAW_ANG;
VEL_X = CONTROL.INPUT.EARTH_VEL(1);
VEL_Y = CONTROL.INPUT.EARTH_VEL(2);
POS_XY = CONTROL.INPUT.EARTH_POS(1:2);
WP_XY = CONTROL.TARGET.MISSION_WAYPOINTS(1:CONTROL.TARGET.MISSION_NUM_WAYPOINTS,2:3)';
NEXT_WP = CONTROL.TARGET.MISSION_COUNT;
M = CONTROL.PARAM.NAV_MPC.PRED_HRZ;
if NEXT_WP == size(WP_XY,2)
    CONTROL.TARGET.NAV_REF_LC(1) = 0;
    CONTROL.TARGET.NAV_REF(1) = 0;
    CONTROL.TARGET.NAV_REF_MPC(1:M,1) = zeros(M,1);
    CONTROL.TARGET.VEL_XY_REF(1) = 0;
    CONTROL.TARGET.VEL_XY_REF(2) = 0;
    CONTROL.TARGET.FORWARD_VEL_REF = 0;
end

%--------------------------------------------------------------
% TRAJECTORY PLANNING
%--------------------------------------------------------------
% x(t) = sum(ai*t^i) i=0...N
% y(t) = sum(bi*t^i) i=0...N
% dx(t)/dt = vx(t) = sum(i*ai*t^(i-1)) i=0...N
% dy(t)/dt = vy(t) = sum(i*bi*t^(i-1)) i=0...N
% Position and distance data
pos_x = [POS_XY(1) WP_XY(1,NEXT_WP:end)]';
pos_y = [POS_XY(2) WP_XY(2,NEXT_WP:end)]'; 
d = abs(diff(pos_x) + 1j*diff(pos_y));
% Delete duplicated points (distance = 0)
ind = find(d>0);
pos_x = [pos_x(ind) ; pos_x(end)];
pos_y = [pos_y(ind) ; pos_y(end)];
d = abs(diff(pos_x) + 1j*diff(pos_y));
% Polynomial parameters
Np = min([4 length(pos_x)+1]);
% Polynomial order
N = Np-1;
% Parameter initialization
a = zeros(Np,1);
b = zeros(Np,1);
a(1) = pos_x(1);
b(1) = pos_y(1);
a(2) = VEL_X;
b(2) = VEL_Y;
% Time vector for target
t_tgt = (1:P)'*tc;
VEL_MAG_TARGET = zeros(P,1);
VEL_ANG_TARGET = zeros(P,1);
% Time matrix for velocity target computation
matTp = zeros(P,N+1);
matTv = zeros(P,N);
for nn = 1:N+1
    matTp(:,nn) = t_tgt.^(nn-1);
end
for nn = 1:N
    matTv(:,nn) = nn*t_tgt.^(nn-1);
end
flag_vel_max = true;
k = 1;
while flag_vel_max
    % Reaching time for the next waypoints
    t = cumsum([0 ; k*sqrt(2)*d(1:N-1)/VEL_MAG_MAX]);    
    % Polynomial coefficient estimation 
    % matBx = matA*a(3:Np);  
    % matBy = matA*b(3:Np)
    matA = zeros(Np-2);
    for nn = 1:Np-2
        matA(:,nn) = t(2:end).^(nn+1);
    end
    matBx = pos_x(2:Np-1) - a(2)*t(2:end) - a(1);
    matBy = pos_y(2:Np-1) - b(2)*t(2:end) - b(1);
    inv_matA = inv(matA);
    a(3:end) = inv_matA*matBx;
    b(3:end) = inv_matA*matBy;
    % Position target calculation
    px_tgt = matTp*a;
    py_tgt = matTp*b; 
    % Magnitude and angle velocity targets calculation
    vx_tgt = matTv*a(2:end);
    vy_tgt = matTv*b(2:end); 
    v_tgt = vx_tgt + 1j*vy_tgt;
    VEL_MAG_TARGET = abs(v_tgt);
    VEL_ANG_TARGET = angle(v_tgt)*(VEL_MAG_TARGET(1)>=0.005) + ...
                    VEL_ANG*ones(size(VEL_ANG_TARGET))*(VEL_MAG_TARGET(1)<0.005);
    % Decreasing velocity factor
    k = k*max(VEL_MAG_TARGET)/VEL_MAG_MAX;
    % Maximun velocity verification
    if (max(VEL_MAG_TARGET)/VEL_MAG_MAX)<=1.01
        flag_vel_max = false;
    end
end

%--------------------------------------------------------------
% UNWRAPPING
%--------------------------------------------------------------
aux1 = VEL_ANG_TARGET(1);
aux2 = VEL_ANG;
INC_VEL_ANG_TARGET = zeros(21,1);
INC_VEL_ANG_TARGET(1) = aux1-aux2;
for nn=1:10
    INC_VEL_ANG_TARGET(2*nn:2*nn+1) = [aux1-aux2-2*nn*pi ; aux1-aux2+2*nn*pi];
end
[~,ind] = min(abs(INC_VEL_ANG_TARGET));
VEL_ANG_TARGET(1) = aux2 + INC_VEL_ANG_TARGET(ind);
for nn = 2:P
    INC_VEL_ANG_TARGET = [VEL_ANG_TARGET(nn)-VEL_ANG_TARGET(nn-1)
                          VEL_ANG_TARGET(nn)-VEL_ANG_TARGET(nn-1)-2*pi
                          VEL_ANG_TARGET(nn)-VEL_ANG_TARGET(nn-1)+2*pi];
    [~,ind] = min(abs(INC_VEL_ANG_TARGET));
    VEL_ANG_TARGET(nn) = VEL_ANG_TARGET(nn-1) + INC_VEL_ANG_TARGET(ind);
end

%--------------------------------------------------------------
% CONTROL BUS UPDATE
%--------------------------------------------------------------
CONTROL.TARGET.NAV_REF_LC(1) = VEL_MAG_TARGET(1);
CONTROL.TARGET.NAV_REF_LC(2) = VEL_ANG_TARGET(1);
if M<=P
    CONTROL.TARGET.NAV_REF_MPC(1:M,1) = VEL_MAG_TARGET(1:M);
    CONTROL.TARGET.NAV_REF_MPC(1:M,2) = VEL_ANG_TARGET(1:M);
else
    CONTROL.TARGET.NAV_REF_MPC(1:M,1) = [VEL_MAG_TARGET(1:P); VEL_MAG_TARGET(end)*ones(M-P,1)];
    CONTROL.TARGET.NAV_REF_MPC(1:M,2) = [VEL_ANG_TARGET(1:P); VEL_ANG_TARGET(end)*ones(M-P,1)];
end
VEL_XY = VEL_MAG_TARGET.*exp(1j*VEL_ANG_TARGET);
CONTROL.TARGET.VEL_XY_REF(1) = real(VEL_XY(1));
CONTROL.TARGET.VEL_XY_REF(2) = imag(VEL_XY(1));
CONTROL.TARGET.NAV_REF = [VEL_MAG_TARGET(1) ; VEL_ANG_TARGET(1)];

return

== matlab function TEST_LIDAR/HARDWARE/COMMUNICATIONS/TCP//IP SLAM/SLAM TX ==
  data: CONTROL input Bus: CONTROL_Bus; PAYLOAD output
function PAYLOAD  = SLAM_CODER(CONTROL)

%--------------------------------------------------------------------------
% INITIALIZATION
%--------------------------------------------------------------------------
persistent init TIMER x y shi
if isempty(init)
    TIMER = 0;
    x = 0;
    y = 0;
    shi = 0;
    init = 1;
end

%--------------------------------------------------------------------------
% TIMER UPDATE
%--------------------------------------------------------------------------
ts = CONTROL.PARAM.SAMPLING_TIME;
TIMER = TIMER + ts;

%--------------------------------------------------------------------------
% FORWARD VELOCITY AND YAW RATE UPDATE
%--------------------------------------------------------------------------
v = CONTROL.INPUT.FORWARD_VELOCITY;
w = CONTROL.INPUT.YAW_RATE;

%--------------------------------------------------------------------------
% INTEGRATION
%--------------------------------------------------------------------------
shi = shi + w*ts;
vx = v*cos(shi);
vy = v*sin(shi);
x = x + vx*ts;
y = y + vy*ts;

if TIMER >= 0.1-ts/2
    % Payload definition
    PAYLOAD = [typecast(single(x),'uint8')'
               typecast(single(y),'uint8')'
               typecast(single(shi),'uint8')'];
    TIMER = 0;
    x = 0;
    y = 0;
    shi = 0;
else
    PAYLOAD = zeros(12,1,'uint8');
end

return
